simulink model "lab4"  (R2023b)
settings: Solver=ode4  StartTime=0.0  StopTime=10.0  FixedStep=2^(-7)  RelTol=1e-3
libraries: simulink x1
settings Model: Creator=insomnia  LastModifiedBy=insomnia

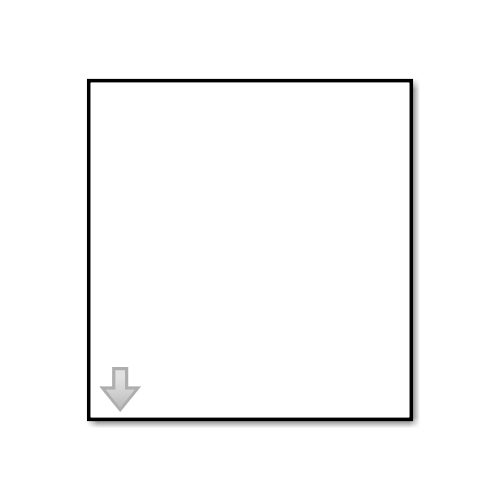
[thumbnail: Simulink's stored preview of the top-level diagram]
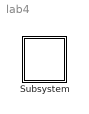
== system lab4 ==
  Subsystem : Subsystem  mask{vx=10, vy=0, x=0, y=5, M=200, R=2, rs=0.2, G=9.81}

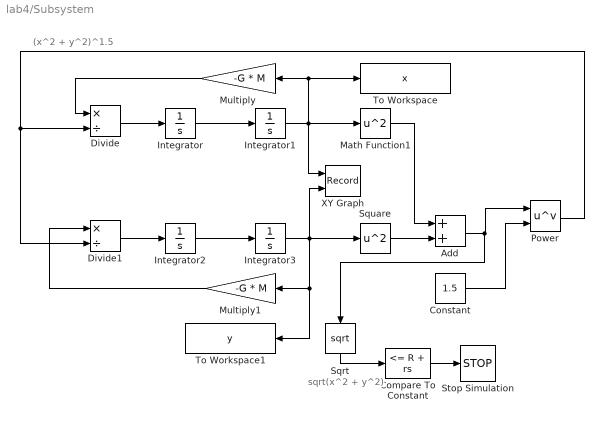
== system lab4/Subsystem ==
  note: sqrt(x^2 + y^2)
  note: (x^2 + y^2)^1.5
  Add : Sum
  Compare To Constant : simulink/Logic and Bit Operations/Compare To Constant  relop=<=  const=R + rs  OutDataTypeStr=boolean
  Constant : Constant  Value=1.5
  Divide : Product  Inputs=*/
  Divide1 : Product  Inputs=*/
  Integrator : Integrator  InitialCondition=vx
  Integrator1 : Integrator  InitialCondition=x
  Integrator2 : Integrator  InitialCondition=vy
  Integrator3 : Integrator  InitialCondition=y
  Math Function1 : Math  Operator=square
  Multiply : Gain  Gain=-G * M
  Multiply1 : Gain  Gain=-G * M
  Power : Math  Operator=pow
  Sqrt : Sqrt
  Square : Math  Operator=square
  Stop Simulation : Stop
  To Workspace : ToWorkspace  VariableName=x  SampleTime=-1
  To Workspace1 : ToWorkspace  VariableName=y  SampleTime=-1
  XY Graph : Record  FileSettingsInternal="{\"entries\":[{\"content\":{\"excelSettings\":{\"content\":{},\"type\":\"Streamout.ExcelSettings\"}},\"type\":\"Streamout.FileSettingStorage\",\"uuid\":\"\"}],\"packageUris\":[\"http:\\/\\/schema.mathworks.com\\/mf0\\/streamout_blocks\\/R2020a\"],\"version\":\"1.0\"}"  Layout=[1 1]  SignalsInternal="{\"entries\":[{\"content\":{\"signals\":[{\"content\":{\"blockPath\":[],\"dimensions\":[1],\"domain\":\"\",\"lineColor\":\"#a2142f\",\"plots\":[ 1 ],\"port\":1,\"sid\":[\"\"],\"signalID\":1,\"signalName\":\"Integrator1\"},\"type\":\"RecordBlkView.Signal\",\"uuid\":\"\"},{\"content\":{\"blockPath\":[],\"dimensions\":[1],\"domain\":\"\",\"lineColor\":\"#139fff\",\"plots\":[ 1 ],\"port\":2,\"sid\":[\"\"],\"signalID\":2,\"signalName\":\"Integrator3\"},\"type\":\"RecordBlkView.Signal\",\"uuid\":\"\"}]},\"type\":\"RecordBlkView.InputSignals\",\"uuid\":\"\"}],\"packageUris\":[\"http:\\/\\/schema.mathworks.com\\/mf0\\/streamout_blocks\\/R2020a\"],\"version\":\"1.0\"}"  VisualizationBindings="{\"xyplotplugin\":{\"info\":[{\"series\":[{\"bindingParametersList\":[{\"parameter\":\"X-Axis\",\"signalID\":1,\"signalName\":\"Integrator1\"},{\"parameter\":\"Y-Axis\",\"signalID\":2,\"signalName\":\"Integrator3\"}],\"seriesID\":0}],\"subplotID\":1}]}}"  CompatibilityTag=XY
  wires:
  Integrator1/1 -> To Workspace/1, Multiply/1, XY Graph/1, Math Function1/1
  Constant/1 -> Power/2
  Multiply/1 -> Divide/1
  Power/1 -> Divide1/2, Divide/2
  Integrator/1 -> Integrator1/1
  Divide1/1 -> Integrator2/1
  Integrator2/1 -> Integrator3/1
  Divide/1 -> Integrator/1
  Integrator3/1 -> To Workspace1/1, Multiply1/1, XY Graph/2, Square/1
  Math Function1/1 -> Add/1
  Multiply1/1 -> Divide1/1
  Square/1 -> Add/2
  Compare To Constant/1 -> Stop Simulation/1
  Sqrt/1 -> Compare To Constant/1
  Add/1 -> Sqrt/1, Power/1
